simulink model "dvbs2transmiter"  (R2025b)
settings: Solver=VariableStepAuto  StartTime=0.0  StopTime=10.0  RelTol=1e-3
undefined symbols (not defined in the file): GenBCHPoly
libraries: commblkcod2 x2, dspsigops x1, commdigbbndpm3 x1, matrix_library x1, commfilt2 x1
settings Model: Creator=Djaga  LastModifiedBy=Djaga

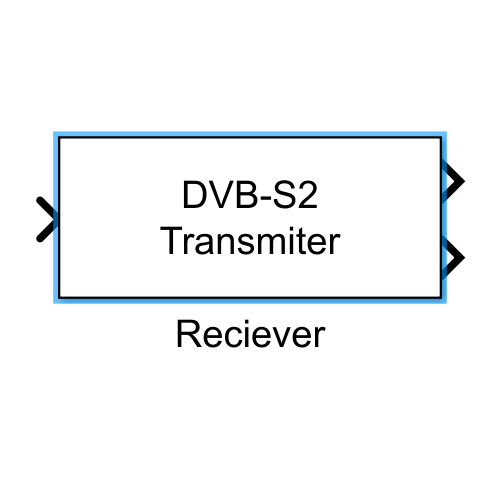
[thumbnail: Simulink's stored preview of the top-level diagram]
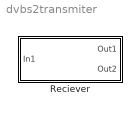
== system dvbs2transmiter ==
  Reciever : Subsystem
      mask Display: disp('DVB-S2\nTransmiter')

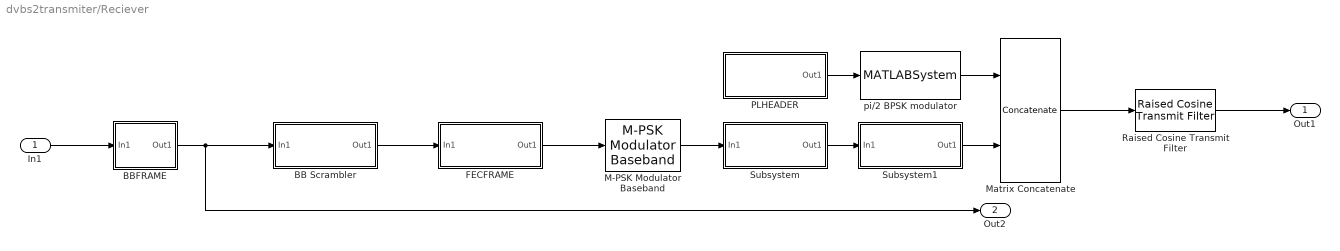
== system dvbs2transmiter/Reciever ==
  In1 : Inport
  BB Scrambler : Subsystem
      mask Display: disp('BB Scrambler')
  BBFRAME : Subsystem
      mask Display: disp('BBFRAME\nBuffering')
  FECFRAME : Subsystem
      mask Display: disp('FEC Encoder')
  M-PSK Modulator Baseband : commdigbbndpm3/M-PSK Modulator Baseband  M=4  InType=Bit  Enc=User-defined  Mapping=[0 2 3 1]  Ph=pi/4  outDtype=double  outWordLen=16  outUDDataType=sfix(16)  outFracLenMode=Best precision  outFracLen=15  outDataTypeStr=double  outLastDataTypeStr=double
  Matrix Concatenate : Concatenate  Mode=Multidimensional array
  PLHEADER : Subsystem
      mask Display: disp('PLНEADER\nGenerator')
  Raised Cosine Transmit Filter : commfilt2/Raised Cosine Transmit Filter  filtType=Square root  R=0.35  filtSpan=10  N=4  filterGain=1  InputProcessing=Columns as channels (frame based)  RateOptions=Enforce single-rate processing  framing=Mute  checkCoeff=off  variableName=rcTxFilt  checkGain=Normalized  sampMode=Mute  saveAsFlag=0  currentFiltSpan=10  D=(10)/2  launchFVT=on  roundingMode=Floor  overflowMode=off  coeffDataTypeStr=Inherit: Same word length as input  coeffMin=[]  coeffMax=[]  coeffLastDataTypeStr=Inherit: Same word length as input  outputDataTypeStr=Inherit: Same as accumulator  outputMin=[]  outputMax=[]  outputLastDataTypeStr=Inherit: Same as accumulator
  Subsystem : Subsystem
      mask Display: disp('Pilot\nInsertion');
  Subsystem1 : Subsystem
      mask Display: disp('PL Scrambler');
  pi/2 BPSK modulator : MATLABSystem  System=Pi2BPSKModulator  InitialPhase=0  SimulateUsing=Code generation
      mask Type: Pi2BPSKModulator
  Out1 : Outport
  Out2 : Outport  Port=2
  wires:
  In1/1 -> BBFRAME/1(In1)
  pi/2 BPSK modulator/1 -> Matrix Concatenate/1
  PLHEADER/1(Out1) -> pi/2 BPSK modulator/1
  Raised Cosine Transmit Filter/1 -> Out1/1
  BBFRAME/1(Out1) -> BB Scrambler/1(In1), Out2/1
  FECFRAME/1(Out1) -> M-PSK Modulator Baseband/1
  Matrix Concatenate/1 -> Raised Cosine Transmit Filter/1
  BB Scrambler/1(Out1) -> FECFRAME/1(In1)
  M-PSK Modulator Baseband/1 -> Subsystem/1(In1)
  Subsystem/1(Out1) -> Subsystem1/1(In1)
  Subsystem1/1(Out1) -> Matrix Concatenate/2

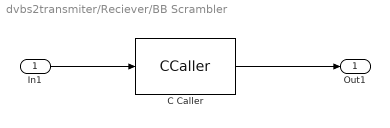
== system dvbs2transmiter/Reciever/BB Scrambler ==
  In1 : Inport
  C Caller : CCaller  FunctionName=bbscrambler  PortSpecificationStruct="%)30     .    V ,   8    (     @         %    \"     (    !     0         %  0 \"0    $    _    07)G3F%M90  4&]R=$YA;64 4V-O<&4     26YD97@     5'EP90      4VEZ90      27-';&]B86P   X    P    !@    @    $          4    (     0    (    !         !   @!U,   #@   #     &    \"     0         !0    @    !     @    $         $  \" '4P   .    .     8    (    !          %    \"     $    %     0         0    !0   $EN<'5T    #@   #@    &    \"     8         !0    @    !     0    $         \"0    @               X    X    !@    @    $          4    (     0    <    !         !     '    8F]O;&5A;@ .    0     8    (    !          %    \"     $    )     0         0    \"0   %LV,S$R+\" Q70         .    ,     8    (    \"0(        %    \"     $    !     0         \"  $       X    P    !@    @    $          4    (     0    (    !         !   @!Y,   #@   #     &    \"     0         !0    @    !     @    $         $  \" 'DP   .    .     8    (    !          %    \"     $    &     0         0    !@   $]U='!U=   #@   #@    &    \"     8         !0    @    !     0    $         \"0    @               X    X    !@    @    $          4    (     0    <    !         !     '    8F]O;&5A;@ .    0     8    (    !          %    \"     $    )     0         0    \"0   %LV,S$R+\" Q70         .    ,     8    (    \"0(        %    \"     $    !     0         \"  $"
  Out1 : Outport
  wires:
  In1/1 -> C Caller/1
  C Caller/1 -> Out1/1

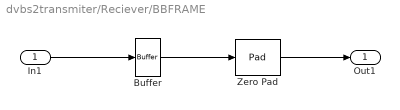
== system dvbs2transmiter/Reciever/BBFRAME ==
  In1 : Inport
  Buffer : Buffer  N=6016  OutputFrames=off
  Zero Pad : dspsigops/Pad  padAlong=Columns  dimsToPad=1  valSrc=Specify via dialog  padVal=0  spec=Output size  padNumOutRowsSpecMethod=User-specified  numOutRows=6312  padNumOutColsSpecMethod=User-specified  numOutCols=1  isVarDimsMode=off  padBeginning=0  padEnd=0  outSizeMode=User-specified  outSize=1  padSigAt=End  trunc_flag=None  roundingMode=Floor  overflowMode=off  truncOrWrapMode=Truncate  wrap_flag=None
  Out1 : Outport  VectorParamsAs1DForOutWhenUnconnected=off
  wires:
  In1/1 -> Buffer/1
  Buffer/1 -> Zero Pad/1
  Zero Pad/1 -> Out1/1

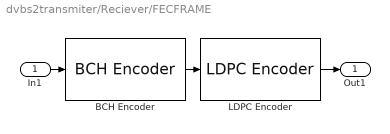
== system dvbs2transmiter/Reciever/FECFRAME ==
  In1 : Inport
  BCH Encoder : commblkcod2/BCH Encoder  n=16383  k=16215  specShortening=on  shortenedK=6312  specGenPoly=on  genPoly=GenBCHPoly(12)  specPrimPoly=off  prPoly='X^4 + X + 1'  specDisableGenCheck=on  specPuncture=off  punctVec=[ones(8,1); zeros(2,1)]
  LDPC Encoder : commblkcod2/LDPC Encoder  ParityCheckMat=LDPC25Matrix
  Out1 : Outport
  wires:
  BCH Encoder/1 -> LDPC Encoder/1
  LDPC Encoder/1 -> Out1/1
  In1/1 -> BCH Encoder/1

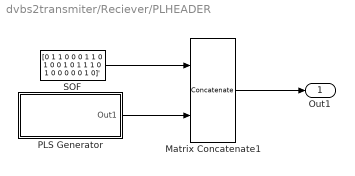
== system dvbs2transmiter/Reciever/PLHEADER ==
  Matrix Concatenate1 : Concatenate  Mode=Multidimensional array
  PLS Generator : Subsystem
      mask Display: disp('PLS\nGenerator')
  SOF : Constant  Value=[0 1 1 0 0 0 1 1 0 1 0 0 1 0 1 1 1 0 1 0 0 0 0 0 1 0]'  VectorParams1D=off  OutDataTypeStr=double
  Out1 : Outport
  wires:
  SOF/1 -> Matrix Concatenate1/1
  PLS Generator/1(Out1) -> Matrix Concatenate1/2
  Matrix Concatenate1/1 -> Out1/1

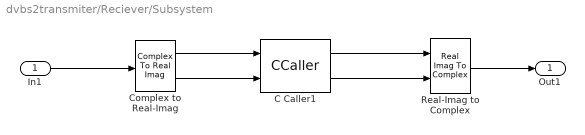
== system dvbs2transmiter/Reciever/Subsystem ==
  In1 : Inport
  C Caller1 : CCaller  FunctionName=pilot_insertion  PortSpecificationStruct="%)30     .    . <   8    (     @         %    \"     0    !     0         %  0 \"0    $    _    07)G3F%M90  4&]R=$YA;64 4V-O<&4     26YD97@     5'EP90      4VEZ90      27-';&]B86P   X    P    !@    @    $          4    (     0    0    !         !  ! !U7W)E#@   #     &    \"     0         !0    @    !    !     $         $  $ '5?<F4.    .     8    (    !          %    \"     $    %     0         0   ...(+2119 chars)"
  Complex to Real-Imag : ComplexToRealImag
  Real-Imag to Complex : RealImagToComplex
  Out1 : Outport
  wires:
  In1/1 -> Complex to Real-Imag/1
  Complex to Real-Imag/1 -> C Caller1/1
  Complex to Real-Imag/2 -> C Caller1/2
  C Caller1/2 -> Real-Imag to Complex/2
  Real-Imag to Complex/1 -> Out1/1
  C Caller1/1 -> Real-Imag to Complex/1

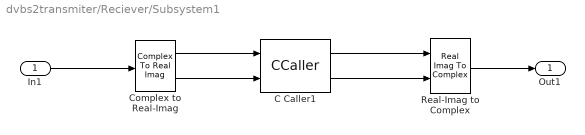
== system dvbs2transmiter/Reciever/Subsystem1 ==
  In1 : Inport
  C Caller1 : CCaller  FunctionName=plscrambler  PortSpecificationStruct="%)30     .    . <   8    (     @         %    \"     0    !     0         %  0 \"0    $    _    07)G3F%M90  4&]R=$YA;64 4V-O<&4     26YD97@     5'EP90      4VEZ90      27-';&]B86P   X    P    !@    @    $          4    (     0    0    !         !  ! !U7W)E#@   #     &    \"     0         !0    @    !    !     $         $  $ '5?<F4.    .     8    (    !          %    \"     $    %     0         0   ...(+2119 chars)"
  Complex to Real-Imag : ComplexToRealImag
  Real-Imag to Complex : RealImagToComplex
  Out1 : Outport
  wires:
  In1/1 -> Complex to Real-Imag/1
  Complex to Real-Imag/1 -> C Caller1/1
  Complex to Real-Imag/2 -> C Caller1/2
  C Caller1/2 -> Real-Imag to Complex/2
  Real-Imag to Complex/1 -> Out1/1
  C Caller1/1 -> Real-Imag to Complex/1

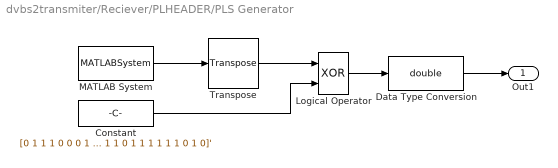
== system dvbs2transmiter/Reciever/PLHEADER/PLS Generator ==
  Constant : Constant  Value=[0 1 1 1 0 0 0 1 1 0 0 1 1 1 0 1 1 0 0 0 0 0 1 1 1 1 0 0 1 0 0 1 0 1 0 1 0 0 1 1 0 1 0 0 0 0 1 0 0 0 1 0 1 1 0 1 1 1 1 1 1 0 1 0]'  OutDataTypeStr=boolean
  Data Type Conversion : DataTypeConversion  OutDataTypeStr=double  SaturateOnIntegerOverflow=off  RndMeth=Floor
  Logical Operator : Logic  Operator=XOR  AllPortsSameDT=off  OutDataTypeStr=boolean
  MATLAB System : MATLABSystem  System=PLS_Codec  InputBits=[ 0, 0, 0, 0, 1, 0, 0 ]  SimulateUsing=Code generation
      mask Type: PLS_Codec
  Transpose : matrix_library/Transpose
  Out1 : Outport
  wires:
  Logical Operator/1 -> Data Type Conversion/1
  Constant/1 -> Logical Operator/2
  MATLAB System/1 -> Transpose/1
  Transpose/1 -> Logical Operator/1
  Data Type Conversion/1 -> Out1/1
